simulink model "shap_momentum_exchange"  (R2018a)
settings: Solver=ode45  StartTime=0.0  StopTime=tf  RelTol=1e-3
values from neighbouring files (symbols this model uses):
  m_drv = 1000    [shapiro_thesis_main.m]
  m_hst = 10000    [shapiro_thesis_main.m]
  r_drv = 10e-3    (= 0.01)    [shapiro_thesis_main.m]
  r_hst = 5e-3    (= 0.005)    [shapiro_thesis_main.m]
undefined symbols (not defined in the file or in its folder): dL, L_tether, n, T
libraries: vrlib x2, aerolibutil x1
settings Model: Creator=jshap  LastModifiedBy=jshap

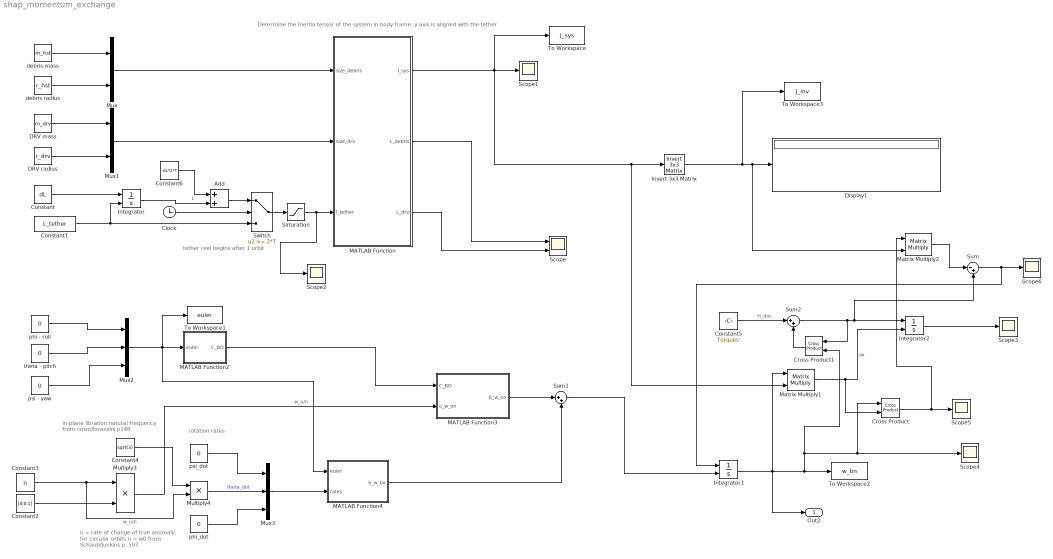
== system shap_momentum_exchange ==
  note: rotation rates
  note: tether reel begins after 1 orbit
  note: Determine the Inertia tensor of the system in body frame. y axis is aligned with the tether
  note: n = rate of change of true anomaly.
      | for circular orbits n = w0
      | from Schaub/Junkins p. 597
  note: in-plane libration natural frequency
      | from cosm/lorenzini p148
  Add : Sum
  Clock : Clock
  Constant : Constant  Value=dL
  Constant1 : Constant  Value=L_tether
  Constant2 : Constant  Value=[0;0;1]
  Constant3 : Constant  Value=n
  Constant4 : Constant  Value=sqrt(3)
  Constant5 : Constant  Value=Torques'  VectorParams1D=off
  Constant6 : Constant  Value=-dL*2*T
  Cross Product : vrlib/Utilities/Cross Product
      settings: SourceProductBaseCode=VR
  Cross Product1 : vrlib/Utilities/Cross Product
      settings: SourceProductBaseCode=VR
  DRV mass : Constant  Value=m_drv
  DRV radius : Constant  Value=r_drv
  Display1 : Display
  Integrator : Integrator  InitialConditionSource=external
  Integrator1 : Integrator  InitialConditionSource=external
  Integrator2 : Integrator  InitialConditionSource=external
  Invert 3x3 Matrix : aerolibutil/Invert  3x3 Matrix
  MATLAB Function : MATLAB Function  TreatAsAtomicUnit=on
  MATLAB Function2 : MATLAB Function  TreatAsAtomicUnit=on
  MATLAB Function3 : MATLAB Function  TreatAsAtomicUnit=on
  MATLAB Function4 : MATLAB Function  TreatAsAtomicUnit=on
  Matrix Multiply1 : Product  Multiplication=Matrix(*)
  Matrix Multiply2 : Product  Multiplication=Matrix(*)
  Multiply3 : Product
  Multiply4 : Product
  Mux : Mux  Inputs=2
  Mux1 : Mux  Inputs=2
  Mux2 : Mux  Inputs=3
  Mux3 : Mux  Inputs=3
  Saturation : Saturate  UpperLimit=50  LowerLimit=0
  Scope : Scope  NumInputPorts=2
  Scope{1..6} (6 alike) : Scope
  Sum : Sum  Inputs=|-+
  Sum1 : Sum  Inputs=|++
  Sum2 : Sum  Inputs=|++
  Switch : Switch  Threshold=2*T  OutMin=0
  To Workspace : ToWorkspace  VariableName=J_sys  SampleTime=-1
  To Workspace1 : ToWorkspace  VariableName=euler  SampleTime=-1
  To Workspace2 : ToWorkspace  VariableName=w_bn  SampleTime=-1
  To Workspace3 : ToWorkspace  VariableName=J_inv  SaveFormat=Timeseries  SampleTime=-1
  "debris mass " : Constant  Value=m_hst
  debris radius : Constant  Value=r_hst
  phi - roll : Constant  Value=0
  phi_dot : Constant  Value=0
  psi - yaw : Constant  Value=0
  psi_dot : Constant  Value=0
  theta - pitch : Constant  Value=0
  Out2 : Outport  SignalName=w_bn
  wires:
  Constant/1 -> Integrator/1
  Constant1/1 -> Integrator/2, Switch/3
  Clock/1 -> Switch/2
  Switch/1 -> Saturation/1
  debris radius/1 -> Mux/2
  "debris mass "/1 -> Mux/1
  Mux/1 -> MATLAB Function/1(size_debris)
  DRV mass/1 -> Mux1/1
  Mux1/1 -> MATLAB Function/2(size_drv)
  DRV radius/1 -> Mux1/2
  MATLAB Function/2(L_debris) -> Scope/1
  MATLAB Function/3(L_drv) -> Scope/2
  theta - pitch/1 -> Mux2/2
  phi - roll/1 -> Mux2/1
  psi - yaw/1 -> Mux2/3
  Mux2/1 -> MATLAB Function4/1(euler), MATLAB Function2/1(euler), To Workspace1/1
  Constant3/1 -> Multiply4/2, Multiply3/1  "w_o/n"
  Constant2/1 -> Multiply3/2
  Multiply3/1 -> MATLAB Function3/2(o_w_on)  "w_o/n"
  Constant4/1 -> Multiply4/1
  Multiply4/1 -> Mux3/2  "theta_dot"
  psi_dot/1 -> Mux3/1
  phi_dot/1 -> Mux3/3
  Mux3/1 -> MATLAB Function4/2(rates)
  MATLAB Function2/1(C_BO) -> MATLAB Function3/1(C_BO)
  MATLAB Function3/1(b_w_on) -> Sum1/1
  MATLAB Function4/1(b_w_bo) -> Sum1/2
  Add/1 -> Switch/1
  Integrator/1 -> Add/2  "L"
  Constant6/1 -> Add/1
  Integrator1/1 -> Matrix Multiply1/1, Out2/1, Cross Product1/2, Cross Product/1, Scope4/1, To Workspace2/1
  Constant5/1 -> Sum2/1  "H_dot"
  Matrix Multiply1/1 -> Cross Product/2, Integrator2/2  "Jw"
  Integrator2/1 -> Scope3/1
  Invert 3x3 Matrix/1 -> To Workspace3/1, Matrix Multiply2/2, Display1/1
  MATLAB Function/1(I_sys) -> To Workspace/1, Matrix Multiply1/2, Invert 3x3 Matrix/1, Scope1/1
  Cross Product/1 -> Matrix Multiply2/1, Scope5/1
  Matrix Multiply2/1 -> Sum/1
  Sum/1 -> Integrator1/1, Scope6/1
  Sum1/1 -> Integrator1/2
  Saturation/1 -> Scope2/1, MATLAB Function/3(l_tether)
  Sum2/1 -> Cross Product1/1, Sum/2, Integrator2/1
  Cross Product1/1 -> Sum2/2

== matlab function shap_momentum_exchange/MATLAB Function ==
  data: size_debris input; I_sys output; size_drv input; l_tether input; L_debris output; L_drv output
function [I_sys,L_debris,L_drv] = dumbbell_inertia(size_debris,size_drv,l_tether)

% Determine system inertia
% Inertia of system in body frame
% y-axis aligned with tether
% 
m_hst = size_debris(1);
r_hst = size_debris(2);

m_drv = size_drv(1);
r_drv = size_drv(2);

%--------- determine mass properties of the system
m_e = (m_drv*m_hst)/(m_drv+m_hst);      % equivalent mass of system (massless tether)

% length of tether from hst to COM
l_hst = (m_drv*l_tether)/(m_hst + m_drv);     % [km]
L_debris = l_hst;
% length of tether from drv to COM
L_drv = l_tether - l_hst;               %[km]

% determine inertial properties
J_hst = endbody_inertia(m_hst,r_hst);
J_drv = endbody_inertia(m_drv,r_drv);

I_sys = [-m_hst*l_hst^2+m_drv*L_drv^2    0   0;...
        0   J_drv(1)-J_hst(1)   0;...
        0   0   -m_hst*l_hst^2+m_drv*L_drv^2];

== matlab function shap_momentum_exchange/MATLAB Function2 ==
  data: euler input; C_BO output
function C_BO = fcn(euler)
phi =euler(1);
theta = euler(2);
psi = euler(3);

C_BO = [cos(theta)*cos(psi) cos(theta)*sin(psi) -sin(theta);...
        sin(phi)*sin(theta)*cos(psi)-cos(phi)*sin(psi) sin(phi)*sin(theta)*sin(psi)+cos(phi)*cos(psi) sin(psi)*cos(theta);...
        cos(phi)*sin(theta)*cos(psi)+sin(phi)*sin(psi) cos(phi)*sin(theta)*sin(psi)-sin(phi)*cos(psi) cos(phi)*cos(theta)];
    
end

== matlab function shap_momentum_exchange/MATLAB Function4 ==
  data: euler input; b_w_bo output; rates input
function b_w_bo = fcn(euler,rates)
phi =euler(1);
theta = euler(2);
psi = euler(3);

%rates = rates*[0; 1; 0];      % only want theta_dot

b_w_bo = [-sin(theta) 0 1;
            sin(phi)*cos(theta) cos(phi) 0;
            cos(phi)*cos(theta) -sin(phi) 0]*rates;

== matlab function shap_momentum_exchange/MATLAB Function3 ==
  data: C_BO input; b_w_on output; o_w_on input
function b_w_on = fcn(C_BO, o_w_on)
%%Determine angular velocity of orbit wrt inertial frame in Body frame
% Jessica Shapiro, Farsai Anantachaisilp, Bianca Lovdahl
% 23 May 2017
% Inputs: (3X1) angular velocity o_w_on, (3X3) DCM: C_BO
%                                     
%outputs: 3x1 b_w_on vector 

%method used: Kinematic Differential equations:
% Vector Basis transformation
% Romano KINEMATICS slide: 14

b_w_on = C_BO*o_w_on; 


end
